simulink model "WarningConditionCalculator"  (R2016b)
settings: Solver=FixedStepAuto  StartTime=0.0  StopTime=10.0  FixedStep=0.1  RelTol=1e-3  EnableMultiTasking=on
undefined symbols (not defined in the file): distanceSensitivity
settings Model: Creator=Josef  LastModifiedBy=takiy
settings OptimizationCC: LifeSpan=inf
settings DebuggingCC: SFUnexpectedBacktrackingDiag=warning  SFNoUnconditionalDefaultTransitionDiag=warning  SFExecutionAtInitializationDiag=none
settings GRTTargetCC: TargetLangStandard=C89/C90 (ANSI)
settings ConfigComp: CovMetricSettings=dw  CovHtmlReporting=on  CovSaveCumulativeToWorkspaceVar=on  CovSaveSingleToWorkspaceVar=on  CovExternalEMLEnable=off

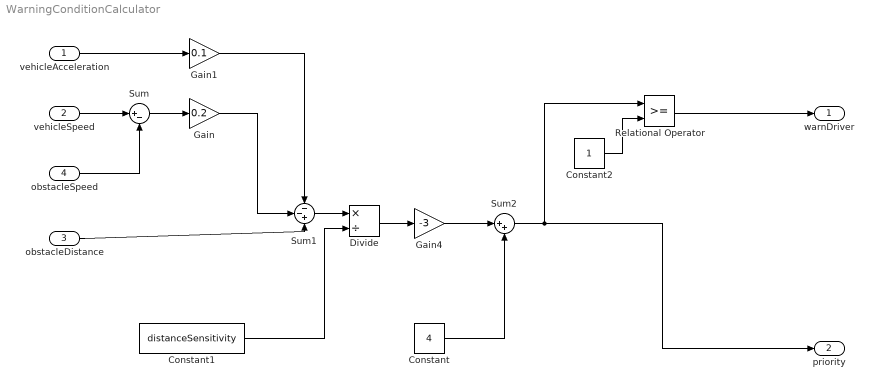
== system WarningConditionCalculator ==
  vehicleAcceleration : Inport
      settings: AttributesFormatString=acceleration
  vehicleSpeed : Inport  Port=2
      settings: AttributesFormatString=speed
  obstacleDistance : Inport  Port=3
      settings: AttributesFormatString=distance
  obstacleSpeed : Inport  Port=4
      settings: AttributesFormatString=speed
  Constant : Constant  Value=4
  Constant1 : Constant  Value=distanceSensitivity
  Constant2 : Constant
  Divide : Product  Inputs=*/
  Gain : Gain  Gain=0.2
  Gain1 : Gain  Gain=0.1
  Gain4 : Gain  Gain=-3
  Relational Operator : RelationalOperator  OutDataTypeStr=boolean  RndMeth=Nearest
  Sum : Sum  Inputs=|+-
  Sum1 : Sum  Inputs=--+
  Sum2 : Sum  Inputs=|++
  warnDriver : Outport
      settings: AttributesFormatString=detectObstacleandWarnDriver
  priority : Outport  Port=2
      settings: AttributesFormatString=signal
  wires:
  Sum/1 -> Gain/1
  vehicleAcceleration/1 -> Gain1/1
  obstacleDistance/1 -> Sum1/3
  Gain/1 -> Sum1/2
  Gain1/1 -> Sum1/1
  vehicleSpeed/1 -> Sum/1
  obstacleSpeed/1 -> Sum/2
  Sum1/1 -> Divide/1
  Constant1/1 -> Divide/2
  Divide/1 -> Gain4/1
  Gain4/1 -> Sum2/1
  Constant/1 -> Sum2/2
  Relational Operator/1 -> warnDriver/1
  Constant2/1 -> Relational Operator/2
  Sum2/1 -> priority/1, Relational Operator/1
